simulink model "lmi_robust_wingrock"  (R2018a)
settings: Solver=VariableStepAuto  StartTime=0.0  StopTime=120.0  RelTol=1e-3
libraries: simulink_extras x3
settings Model: Creator=saad  LastModifiedBy=saad

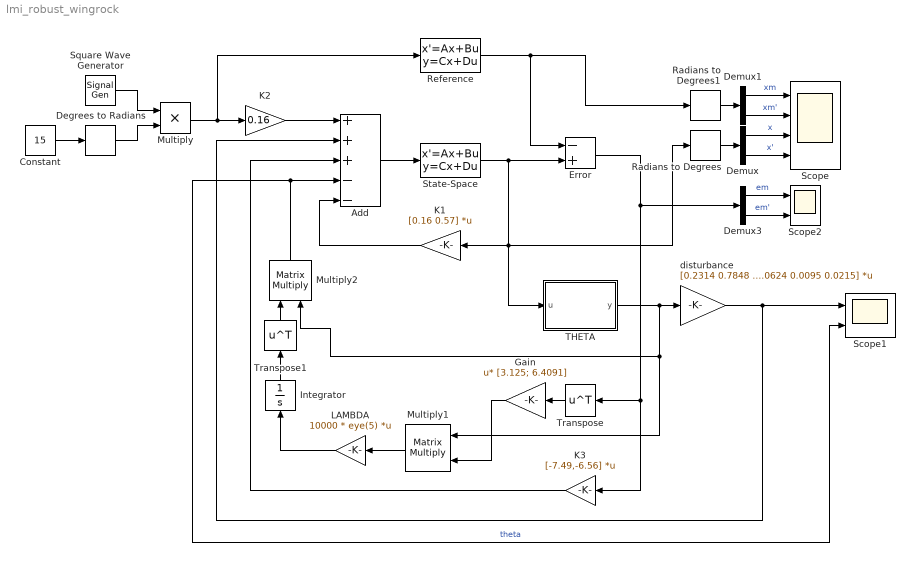
== system lmi_robust_wingrock ==
  Add : Sum  Inputs=+++--
  Constant : Constant  Value=15
  Degrees to Radians : simulink_extras/Transformations/Degrees to Radians
  Demux : Demux  Outputs=2
  Demux1 : Demux  Outputs=2
  Demux3 : Demux  Outputs=2
  Error : Sum  Inputs=-+
  Gain : Gain  Gain=[3.125; 6.4091]  Multiplication=Matrix(u*K)
  Integrator : Integrator
  K1 : Gain  Gain=[0.16 0.57]  Multiplication=Matrix(K*u)
  K2 : Gain  Gain=0.16
  K3 : Gain  Gain=[-7.49,-6.56]  Multiplication=Matrix(K*u)
  LAMBDA : Gain  Gain=10000 * eye(5)  Multiplication=Matrix(K*u)
  Multiply : Product
  Multiply1 : Product  Multiplication=Matrix(*)
  Multiply2 : Product  Multiplication=Matrix(*)
  Radians to Degrees : simulink_extras/Transformations/Radians to Degrees
  Radians to Degrees1 : simulink_extras/Transformations/Radians to Degrees
  Reference : StateSpace  A=[0 1;-0.16 -0.5656]  B=[0;0.16]  C=eye(2)  D=[0;0]  InitialCondition=0  ContinuousStateAttributes={'angle', 'angular_speed'}
  Scope : Scope  NumInputPorts=4
  Scope1 : Scope  NumInputPorts=2
  Scope2 : Scope  NumInputPorts=2
  Square Wave Generator : SignalGenerator  WaveForm=square  Amplitude=-1  Frequency=pi/30  Units=rad/sec
  State-Space : StateSpace  A=[0 1;0 0]  B=[0;1]  C=eye(2)  D=[0;0]  InitialCondition=0  ContinuousStateAttributes={'angle', 'angular_speed'}
  THETA : MATLAB Function  TreatAsAtomicUnit=on
  Transpose : Math  Operator=transpose  SaturateOnIntegerOverflow=on
  Transpose1 : Math  Operator=transpose  SaturateOnIntegerOverflow=on
  disturbance : Gain  Gain=[0.2314 0.7848 -0.0624 0.0095 0.0215]  Multiplication=Matrix(K*u)
  wires:
  Constant/1 -> Degrees to Radians/1
  Square Wave Generator/1 -> Multiply/1
  Degrees to Radians/1 -> Multiply/2
  Add/1 -> State-Space/1
  Multiply/1 -> Reference/1, K2/1
  K2/1 -> Add/1
  Reference/1 -> Error/1, Radians to Degrees1/1
  State-Space/1 -> Error/2, THETA/1(u), Radians to Degrees/1, K1/1
  Demux/1 -> Scope/3  "x"
  Demux/2 -> Scope/4  "x'"
  Radians to Degrees/1 -> Demux/1
  Demux1/1 -> Scope/1  "xm"
  Demux1/2 -> Scope/2  "xm'"
  Radians to Degrees1/1 -> Demux1/1
  THETA/1(y) -> disturbance/1, Multiply2/2, Multiply1/1
  disturbance/1 -> Add/2, Scope1/1
  Transpose/1 -> Gain/1
  Gain/1 -> Multiply1/2
  Multiply1/1 -> LAMBDA/1
  LAMBDA/1 -> Integrator/1
  Integrator/1 -> Transpose1/1
  Transpose1/1 -> Multiply2/1
  K1/1 -> Add/5
  Multiply2/1 -> Scope1/2, Add/4  "theta"
  K3/1 -> Add/3
  Demux3/2 -> Scope2/2  "em'"
  Demux3/1 -> Scope2/1  "em"
  Error/1 -> Demux3/1, K3/1, Transpose/1

== matlab function lmi_robust_wingrock/THETA ==
  data: u input; y output
function y = fcn(u)

    y = [u(1); u(2); abs(u(1))*u(2); abs(u(2))*u(2); u(1)^3];
